simulink model "nn_template"  (R2014a)
settings: Solver=FixedStepDiscrete  StartTime=0.0  StopTime=inf  FixedStep=SampleTime  RelTol=1e-3
libraries: dspbuff3 x1, dspmtrx3 x1
settings Model: Creator=georg  LastModifiedBy=georg

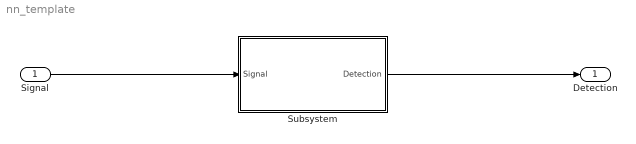
== system nn_template ==
  Signal : Inport
  Subsystem : Subsystem
  Detection : Outport
  wires:
  Signal/1 -> Subsystem/1(Signal)
  Subsystem/1(Detection) -> Detection/1

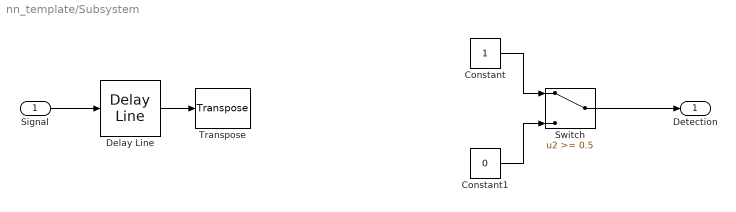
== system nn_template/Subsystem ==
  Signal : Inport
  Constant : Constant
  Constant1 : Constant  Value=0
  Delay Line : dspbuff3/Delay Line  siz=2  ic=0  directfeed=off  enable_output=off  hold_output=off  TreatMby1Signals=One channel
  Switch : Switch  Threshold=0.5
  Transpose : dspmtrx3/Transpose  Hermitian=off  overflowFlag=off
  Detection : Outport
  wires:
  Switch/1 -> Detection/1
  Constant/1 -> Switch/1
  Constant1/1 -> Switch/3
  Delay Line/1 -> Transpose/1
  Signal/1 -> Delay Line/1
